simulink model "comm_projectC"  (R2020b)
settings: Solver=VariableStepAuto  StartTime=0.0  StopTime=0.002  RelTol=1e-3
libraries: commanapbnd3 x2
settings Model: Creator=khale  LastModifiedBy=khale

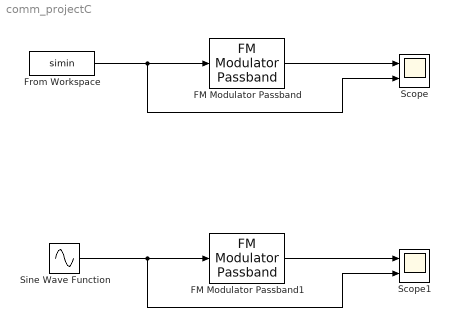
== system comm_projectC ==
  FM Modulator Passband : commanapbnd3/FM Modulator Passband  Fc=10000  Ph=0  Kc=kf
      settings: SourceProductBaseCode=CM
  FM Modulator Passband1 : commanapbnd3/FM Modulator Passband  Fc=10000  Ph=0  Kc=kf
      settings: SourceProductBaseCode=CM
  From Workspace : FromWorkspace  VariableName=simin  SampleTime=0.0000001
  Scope : Scope  NumInputPorts=2
  Scope1 : Scope  NumInputPorts=2
  Sine Wave Function : Sin  Amplitude=1.5  Frequency=2*pi*2000  SampleTime=0.0000001
  wires:
  From Workspace/1 -> Scope/2, FM Modulator Passband/1
  FM Modulator Passband/1 -> Scope/1
  Sine Wave Function/1 -> Scope1/2, FM Modulator Passband1/1
  FM Modulator Passband1/1 -> Scope1/1
